simulink model "circuit"  (R2022b)
settings: Solver=VariableStepAuto  StartTime=0.0  StopTime=30  RelTol=1e-3
libraries: fuzblock x1
settings Model: Creator=andre  LastModifiedBy=Paulo Cortesão

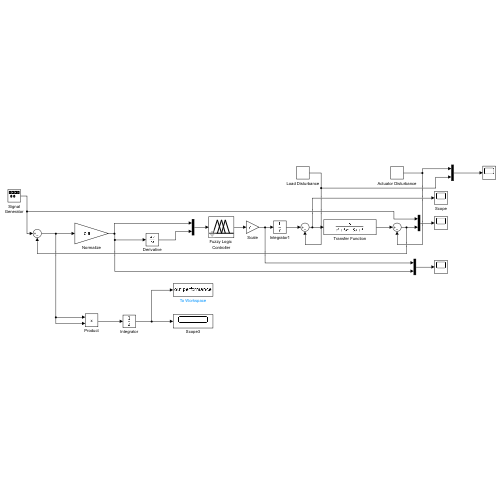
[thumbnail: Simulink's stored preview of the top-level diagram]
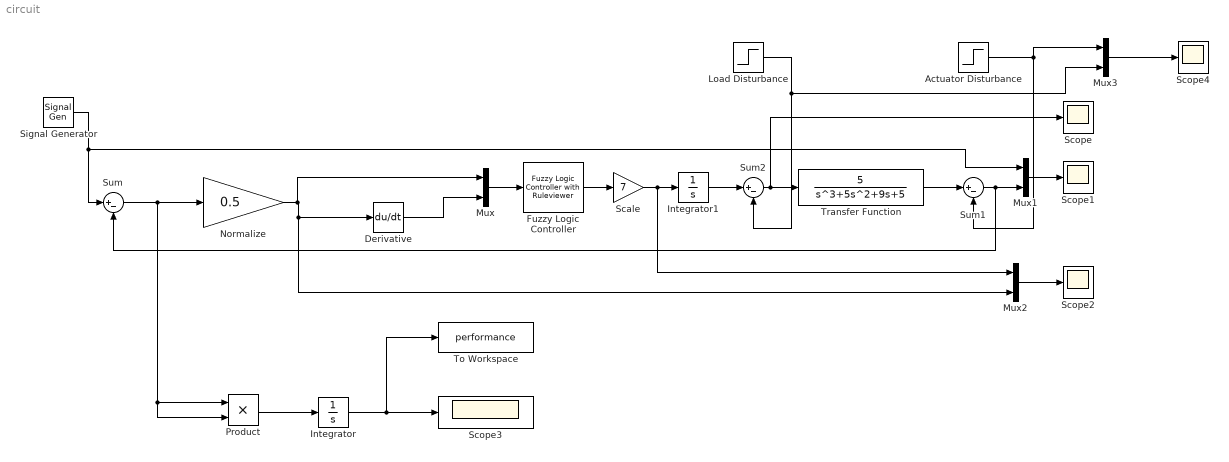
== system circuit ==
  Actuator Disturbance : Step  SampleTime=0
  Derivative : Derivative
  Fuzzy Logic Controller : fuzblock/Fuzzy Logic  Controller  with Ruleviewer  fismatrix=io_3_mamdani  Ts=2
  Integrator : Integrator
  Integrator1 : Integrator
  Load Disturbance : Step  SampleTime=0
  Mux{,1..3} (4 alike) : Mux  Inputs=2
  Normalize : Gain  Gain=0.5
  Product : Product
  Scale : Gain  Gain=7
  Scope{,1..4} (5 alike) : Scope
  Signal Generator : SignalGenerator  Units=rad/sec
  Sum : Sum  Inputs=|+-
  Sum1 : Sum  Inputs=|+-
  Sum2 : Sum  Inputs=|+-
  To Workspace : ToWorkspace  VariableName=performance  SaveFormat=Timeseries  SampleTime=-1
  Transfer Function : TransferFcn  Numerator=[5]  Denominator=[1 5 9 5]
  wires:
  Signal Generator/1 -> Mux1/1, Sum/1
  Sum/1 -> Product/1, Product/2, Normalize/1
  Normalize/1 -> Mux/1, Mux2/2, Derivative/1
  Derivative/1 -> Mux/2
  Scale/1 -> Mux2/1, Integrator1/1
  Mux/1 -> Fuzzy Logic Controller/1
  Fuzzy Logic Controller/1 -> Scale/1
  Integrator1/1 -> Sum2/1
  Load Disturbance/1 -> Mux3/2, Sum2/2
  Sum2/1 -> Scope/1, Transfer Function/1
  Transfer Function/1 -> Sum1/1
  Actuator Disturbance/1 -> Mux3/1, Sum1/2
  Mux1/1 -> Scope1/1
  Sum1/1 -> Sum/2, Mux1/2
  Mux2/1 -> Scope2/1
  Product/1 -> Integrator/1
  Integrator/1 -> To Workspace/1, Scope3/1
  Mux3/1 -> Scope4/1
